simulink model "AirRefueling_Platform_IBVS"  (R2022b)
settings: Solver=ode4  StartTime=0.0  StopTime=60  FixedStep=0.01  RelTol=1e-5  AbsTol=1e-4  EnableMultiTasking=on
InitFcn:
  | F16_Init
values from neighbouring files (symbols this model uses):
  airSpeed = 393.72    [F16_Init.m]
  alpha0 = trimAlpha*180/pi    (= 6.62393794015)    [F16_Init.m]
  altitude = 9843    [F16_Init.m]
  b_ref = 30.0    (= 30)    [F16_Init.m]
  C2m = [C(1,:) ... (first row only)    [F16_Init.m]
  Cdr_ = 0.8    [hose_parameter4dock.mat]
  d_f_rc = [4.45;0;-3.81]    [F16_Init.m]
  d_pr_cam = d_pr_rc - d_cam_rc    [F16_Init.m]
  d_pr_rc = [8.2;0.45;-3.3]    [F16_Init.m]
  dLEF = 0    [F16_Init.m]
  dtheta10 = [0 0 0 0 0 0 0 0 0 0]    [hose_parameter4dock.mat]
  dtheta20 = [0 0 0 0 0 0 0 0 0 0]    [hose_parameter4dock.mat]
  fi_flag = 1    [F16_Init.m]
  height = 3000    [hose_parameter4dock.mat]
  k_reel = 0.5    [hose_parameter4dock.mat]
  Kc = [ ... (first row only)    [F16_Init.m]
  kd = 500    [hose_parameter4dock.mat]
  Ki = zeros(4,3)    [F16_Init.m]
  Kp = zeros(4,18)    [F16_Init.m]
  l0 = 1.44444444444    [hose_parameter4dock.mat]
  l1 = 2    [hose_parameter4dock.mat]
  l_density = 4.1    [hose_parameter4dock.mat]
  m0 = 5.92222222222    [hose_parameter4dock.mat]
  mass = 636.94    [F16_Init.m]
  Mdr = 29.5    [hose_parameter4dock.mat]
  N = 10    [hose_parameter4dock.mat]
  p0_rc = [-30.7;1;10]    [F16_Init.m]
  Rdr = 0.305    [hose_parameter4dock.mat]
  Rl = 0.0336    [hose_parameter4dock.mat]
  T_reel_initial = 1610    [hose_parameter4dock.mat]
  theta10 = [0.459903280115 0.432776206681 0.412025416789 0.390288667864 0.365355881715 0.340009787283 0.310854701374 0.281345523746 0.248396428993 0.214590627751]    [hose_parameter4dock.mat]
  theta20 = [0 0 0 0 0 0 0 0 0 0]    [hose_parameter4dock.mat]
  trim_ail = 0.00874607850103852    (= 0.00874607850104)    [F16_Init.m]
  trim_control = [trim_thrust;trim_ele;trim_ail;trim_rud]    [F16_Init.m]
  trim_ele = -2.97973164860638    (= -2.97973164861)    [F16_Init.m]
  trim_rud = 0.0680302158182712    (= 0.0680302158183)    [F16_Init.m]
  trim_state1 = [trim_state;0;0;0;0;0;0]    [F16_Init.m]
  trim_thrust = 2279.08519954656    (= 2279.08519955)    [F16_Init.m]
  visual_err = [0;0;0]    [F16_Init.m]
  vt0 = [120 0 0]    [hose_parameter4dock.mat]
undefined symbols (not defined in the file or in its folder): F, MIL, STD
libraries: etargetslib x11, dspnetwork x10, aerolibconvert2 x4, aerolibasang x4, simulink x2, aerolibatmos2 x2, aerolibwind2 x2, aerolibobsolete x2, aerolibadyn x1, aerolibanimutils x1, slrealtimeiplib x1
(part 2 of 3)

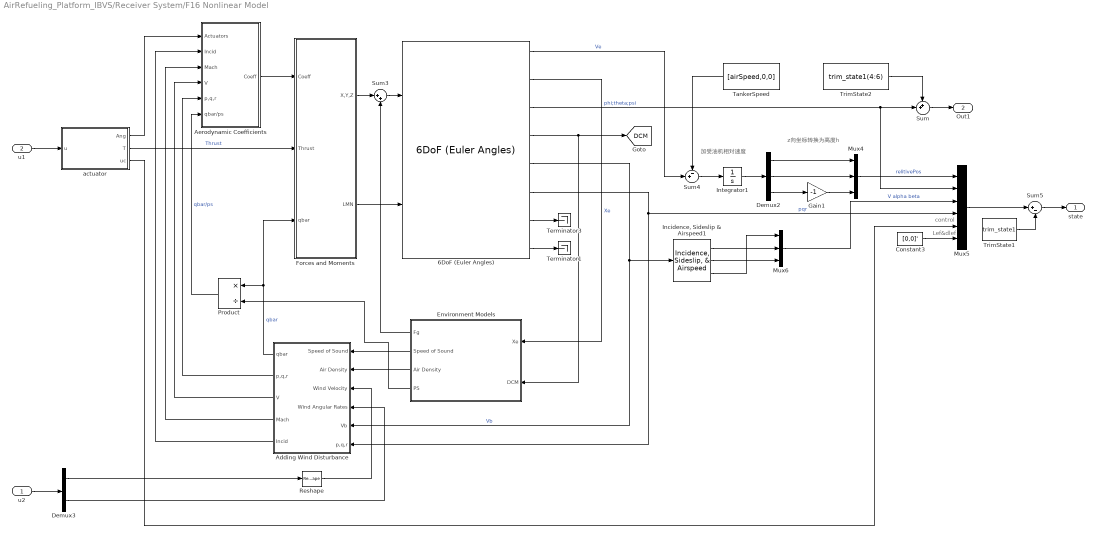
== system AirRefueling_Platform_IBVS/Receiver System/F16 Nonlinear Model ==
  note: 加受油机相对速度
  note: z向坐标转换为高度h
  note: Lef&dlef
  note: control
  u2 : Inport
  u1 : Inport  Port=2
  6DoF (Euler Angles) : aerolibobsolete/6DoF (Euler Angles)  units=English (Velocity in ft/s)  mtype=Fixed  rep=Euler Angles  xme_0=xyz_0  Vm_0=uvw_0  eul_0=Euler_0  pm_0=pqr_0  mass_0=mass  mass_e=0.5  mass_f=2.0  inertia=Inertia  inertia_e=eye(3)  inertia_f=2*eye(3)  k_quat=1.0
  Adding Wind Disturbance : Subsystem
  Aerodynamic Coefficients : Subsystem
  Constant3 : Constant  Value=[0,0]'
  Demux2 : Demux  Outputs=3
  Demux3 : Demux  Outputs=2
  Environment Models : Subsystem
  Forces and Moments : Subsystem
  Gain1 : Gain  Gain=-1
  "Incidence, Sideslip & Airspeed1" : aerolibasang/Incidence, Sideslip, & Airspeed
  Integrator1 : Integrator
  Mux4 : Mux  Inputs=3
  Mux5 : Mux  Inputs=6
  Mux6 : Mux  Inputs=3
  Product : Product  Inputs=*/  InputSameDT=on  SaturateOnIntegerOverflow=on  OutDataTypeStr=Inherit: Same as first input
  Reshape : Reshape
  Sum : Sum  Inputs=++|
  Sum3 : Sum  Inputs=|++  InputSameDT=on  SaturateOnIntegerOverflow=on  OutDataTypeStr=Inherit: Same as first input
  Sum4 : Sum  Inputs=-+|
  Sum5 : Sum  Inputs=|+-
  TankerSpeed : Constant  Value=[airSpeed,0,0]
  Terminator1 : Terminator
  Terminator3 : Terminator
  TrimState1 : Constant  Value=trim_state1
  TrimState2 : Constant  Value=trim_state1(4:6)
  actuator : Subsystem
  state : Outport
  Out1 : Outport  Port=2
  tag scope: DCM=global
  wires:
  6DoF (Euler Angles)/8 -> Terminator1/1
  6DoF (Euler Angles)/7 -> Terminator3/1
  6DoF (Euler Angles)/4 -> Environment Models/2(DCM), [DCM]
  Adding Wind Disturbance/5(Incid) -> Aerodynamic Coefficients/2(Incid)
  Aerodynamic Coefficients/1(Coeff) -> Forces and Moments/1(Coeff)
  Environment Models/2(Speed of Sound) -> Adding Wind Disturbance/1(Speed of Sound)
  Environment Models/3(Air Density) -> Adding Wind Disturbance/2(Air Density)
  Forces and Moments/2(LMN) -> 6DoF (Euler Angles)/2
  Adding Wind Disturbance/1(qbar) -> Forces and Moments/3(qbar), Product/1  "qbar"
  Forces and Moments/1(X,Y,Z) -> Sum3/1
  Sum3/1 -> 6DoF (Euler Angles)/1
  Environment Models/1(Fg) -> Sum3/2
  Adding Wind Disturbance/3(V) -> Aerodynamic Coefficients/4(V)
  Adding Wind Disturbance/4(Mach) -> Aerodynamic Coefficients/3(Mach)
  Adding Wind Disturbance/2("p,q,r ") -> Aerodynamic Coefficients/5(p,q,r)
  Environment Models/4(PS) -> Product/2
  Product/1 -> Aerodynamic Coefficients/6(qbar/ps)  "qbar/ps"
  u1/1 -> actuator/1(u)
  actuator/2(T) -> Forces and Moments/2(Thrust)  "Thrust"
  actuator/1(Ang) -> Aerodynamic Coefficients/1(Actuators)
  6DoF (Euler Angles)/3 -> Mux5/2, Sum/2  "phi;theta;psi"
  "Incidence, Sideslip & Airspeed1"/1 -> Mux6/2
  "Incidence, Sideslip & Airspeed1"/2 -> Mux6/3
  Mux6/1 -> Mux5/3  "V alpha beta"
  "Incidence, Sideslip & Airspeed1"/3 -> Mux6/1
  6DoF (Euler Angles)/6 -> Adding Wind Disturbance/6(p,q,r), Mux5/4  "pqr"
  6DoF (Euler Angles)/5 -> Adding Wind Disturbance/5(Vb), "Incidence, Sideslip & Airspeed1"/1  "Vb"
  Mux5/1 -> Sum5/1
  TrimState1/1 -> Sum5/2
  Sum5/1 -> state/1
  actuator/3(uc) -> Mux5/5
  Constant3/1 -> Mux5/6
  Demux2/2 -> Mux4/2
  Demux2/3 -> Gain1/1
  Mux4/1 -> Mux5/1  "relitivePos"
  Demux2/1 -> Mux4/1
  Gain1/1 -> Mux4/3
  Sum4/1 -> Integrator1/1
  Integrator1/1 -> Demux2/1
  6DoF (Euler Angles)/2 -> Environment Models/1(Xe)  "Xe"
  u2/1 -> Demux3/1
  Reshape/1 -> Adding Wind Disturbance/3(Wind Velocity)
  Demux3/1 -> Reshape/1
  Sum/1 -> Out1/1
  Demux3/2 -> Adding Wind Disturbance/4(Wind Angular Rates)
  TrimState2/1 -> Sum/1
  6DoF (Euler Angles)/1 -> Sum4/2  "Ve"
  TankerSpeed/1 -> Sum4/1

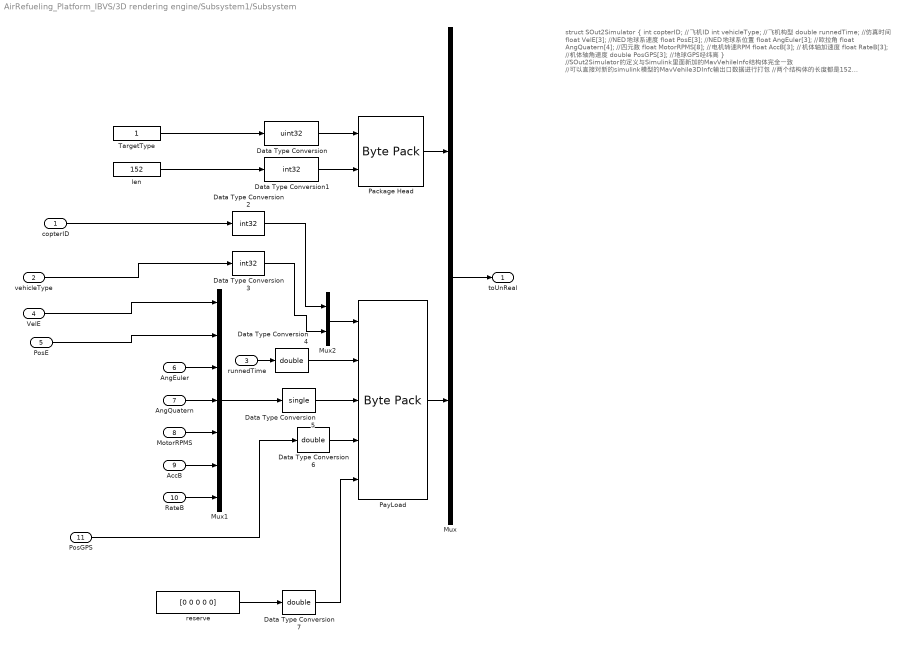
== system AirRefueling_Platform_IBVS/3D rendering engine/Subsystem1/Subsystem ==
  note: struct SOut2Simulator
      | {
      | int copterID; //飞机ID
      | int vehicleType; //飞机构型
      | double runnedTime; //仿真时间
      | float VelE[3]; //NED地球系速度
      | float PosE[3]; //NED地球系位置
      | float AngEuler[3]; //欧拉角
      | float AngQuatern[4]; //四元数
      | float MotorRPMS[8]; //电机转速RPM
      | float AccB[3]; //机体轴加速度
      | float RateB[3]; //机体轴角速度
      | double PosGPS[3]; //地球GPS经纬高
      | }
      |
      | //SOut2Simulator的定义与Simulink里面新加的MavVehileInfo结构体完全一致
      | //可以直接对新的simulink模型的MavVehile3DInfo输出口数据进行打包
      | //两个结构体的长度都是152
      | sizeof(SOut2Simulator) = sizeof(MavVehileInfo) = 152
      |
      | 打包封装的结构体为
      | typedef struct _netDataShort
      | {
      | TargetType tg; //这里目前随便填，写1即可 uint32
      | int len; //这个长度为传输结构体长度，目前是152
      | char payload[192]; //这里面前152位存放了SOut2Simulator结构体数据，后面的40位保留
      | }netDataShort;
      |
      | //UDP包的总长度为200
      | sizeof(netDataShort) = 200
      |
      | //发送的UDP端口号为：20010
  copterID : Inport  PortDimensions=1
  vehicleType : Inport  Port=2  PortDimensions=1
  runnedTime : Inport  Port=3  PortDimensions=1
  "VelE " : Inport  Port=4  PortDimensions=3
  PosE : Inport  Port=5  PortDimensions=3
  AngEuler : Inport  Port=6  PortDimensions=3
  AngQuatern : Inport  Port=7  PortDimensions=4
  MotorRPMS : Inport  Port=8  PortDimensions=8
  AccB : Inport  Port=9  PortDimensions=3
  RateB : Inport  Port=10  PortDimensions=3
  PosGPS : Inport  Port=11  PortDimensions=3
  Data Type Conversion : DataTypeConversion  OutDataTypeStr=uint32  SaturateOnIntegerOverflow=off  RndMeth=Floor
  Data Type Conversion1 : DataTypeConversion  OutDataTypeStr=int32  SaturateOnIntegerOverflow=off  RndMeth=Floor
  Data Type Conversion2 : DataTypeConversion  OutDataTypeStr=int32  SaturateOnIntegerOverflow=off  RndMeth=Floor
  Data Type Conversion3 : DataTypeConversion  OutDataTypeStr=int32  SaturateOnIntegerOverflow=off  RndMeth=Floor
  Data Type Conversion4 : DataTypeConversion  OutDataTypeStr=double  SaturateOnIntegerOverflow=off  RndMeth=Floor
  Data Type Conversion5 : DataTypeConversion  OutDataTypeStr=single  SaturateOnIntegerOverflow=off  RndMeth=Floor
  Data Type Conversion6 : DataTypeConversion  OutDataTypeStr=double  SaturateOnIntegerOverflow=off  RndMeth=Floor
  Data Type Conversion7 : DataTypeConversion  OutDataTypeStr=double  SaturateOnIntegerOverflow=off  RndMeth=Floor
  Mux : Mux  Inputs=2
  Mux1 : Mux  Inputs=7
  Mux2 : Mux  Inputs=2
  Package Head : etargetslib/Byte Pack  datatypes={'uint32','int32'}  byteAlign=4
  PayLoad : etargetslib/Byte Pack  datatypes={'int32','double','single','double','double'}  byteAlign=8
  TargetType : Constant  OutDataTypeStr=Inherit: Inherit via back propagation
  len : Constant  Value=152  OutDataTypeStr=Inherit: Inherit via back propagation
  reserve : Constant  Value=[0 0 0 0 0]  OutDataTypeStr=double
  toUnReal : Outport  VectorParamsAs1DForOutWhenUnconnected=off
  wires:
  runnedTime/1 -> Data Type Conversion4/1
  RateB/1 -> Mux1/7
  PayLoad/1 -> Mux/2
  "VelE "/1 -> Mux1/1
  Mux1/1 -> Data Type Conversion5/1
  PosGPS/1 -> Data Type Conversion6/1
  Package Head/1 -> Mux/1
  AccB/1 -> Mux1/6
  Mux/1 -> toUnReal/1
  MotorRPMS/1 -> Mux1/5
  AngQuatern/1 -> Mux1/4
  copterID/1 -> Data Type Conversion2/1
  len/1 -> Data Type Conversion1/1
  vehicleType/1 -> Data Type Conversion3/1
  PosE/1 -> Mux1/2
  TargetType/1 -> Data Type Conversion/1
  reserve/1 -> Data Type Conversion7/1
  Mux2/1 -> PayLoad/1
  AngEuler/1 -> Mux1/3
  Data Type Conversion5/1 -> PayLoad/3
  Data Type Conversion2/1 -> Mux2/1
  Data Type Conversion1/1 -> Package Head/2
  Data Type Conversion6/1 -> PayLoad/4
  Data Type Conversion/1 -> Package Head/1
  Data Type Conversion3/1 -> Mux2/2
  Data Type Conversion4/1 -> PayLoad/2
  Data Type Conversion7/1 -> PayLoad/5

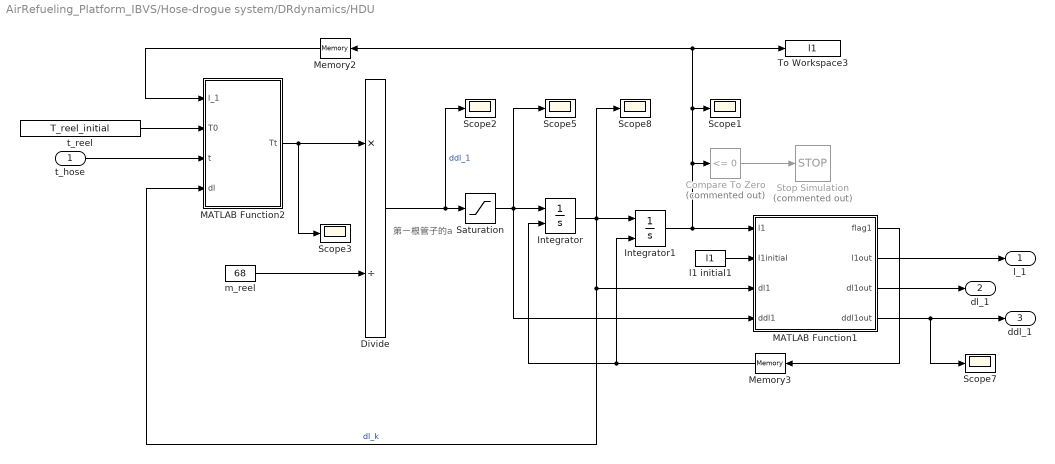
== system AirRefueling_Platform_IBVS/Hose-drogue system/DRdynamics/HDU ==
  note: 第一根管子的a
  t_hose : Inport
  Compare To Zero : simulink/Logic and Bit Operations/Compare To Zero  Commented=on  relop=<=  OutDataTypeStr=boolean
  Divide : Product  Inputs=*/
  Integrator : Integrator  ExternalReset=rising  UpperSaturationLimit=0.3  LowerSaturationLimit=-0.3
  Integrator1 : Integrator  ExternalReset=rising  InitialCondition=l1
  MATLAB Function1 : MATLAB Function  TreatAsAtomicUnit=on
  MATLAB Function2 : MATLAB Function  TreatAsAtomicUnit=on
  Memory2 : Memory  InitialCondition=l1
  Memory3 : Memory
  Saturation : Saturate  UpperLimit=3  LowerLimit=-3
  Scope{1..3,5,7..8} (6 alike) : Scope
  Stop Simulation : Stop  Commented=on
  To Workspace3 : ToWorkspace  VariableName=l1  SampleTime=-1
  l1 initial1 : Constant  Value=l1
  m_reel : Constant  Value=68
  t_reel : Constant  Value=T_reel_initial
  l_1 : Outport
  dl_1 : Outport  Port=2
  ddl_1 : Outport  Port=3
  wires:
  MATLAB Function2/1(Tt) -> Scope3/1, Divide/1
  m_reel/1 -> Divide/2
  Divide/1 -> Saturation/1, Scope2/1  "ddl_1"
  Integrator/1 -> Integrator1/1, MATLAB Function1/3(dl1), MATLAB Function2/4(dl), Scope8/1  "dl_k"
  Saturation/1 -> MATLAB Function1/4(ddl1), Integrator/1, Scope5/1
  t_reel/1 -> MATLAB Function2/2(T0)
  Compare To Zero/1 -> Stop Simulation/1
  l1 initial1/1 -> MATLAB Function1/2(l1initial)
  MATLAB Function1/4(ddl1out) -> Scope7/1, ddl_1/1
  MATLAB Function1/1(flag1) -> Memory3/1
  Memory2/1 -> MATLAB Function2/1(l_1)
  Memory3/1 -> Integrator/2, Integrator1/2
  Integrator1/1 -> MATLAB Function1/1(l1), Compare To Zero/1, To Workspace3/1, Memory2/1, Scope1/1
  MATLAB Function1/2(l1out) -> l_1/1
  MATLAB Function1/3(dl1out) -> dl_1/1
  t_hose/1 -> MATLAB Function2/3(t)

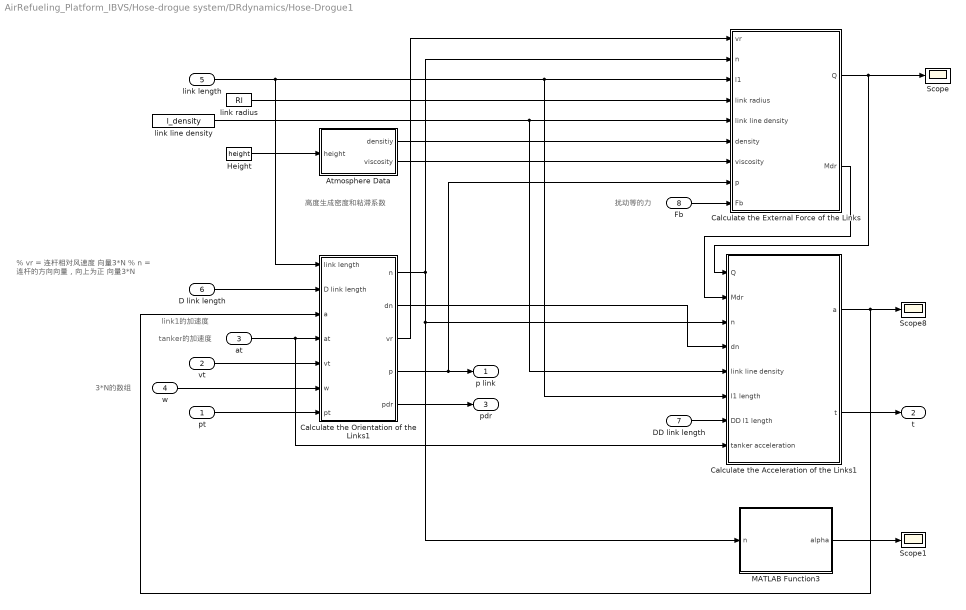
== system AirRefueling_Platform_IBVS/Hose-drogue system/DRdynamics/Hose-Drogue1 ==
  note: % vr = 连杆相对风速度 向量3*N
      | % n = 连杆的方向向量，向上为正 向量3*N
  note: link1的加速度
  note: tanker的加速度
  note: 3*N的数组
  note: 扰动等的力
  note: 高度生成密度和粘滞系数
  pt : Inport
  vt : Inport  Port=2
  at : Inport  Port=3
  w : Inport  Port=4
  link length : Inport  Port=5
  D link length : Inport  Port=6
  DD link length : Inport  Port=7
  Fb : Inport  Port=8
  Atmosphere Data : Subsystem
  Calculate the Acceleration of the Links1 : Subsystem
  Calculate the External Force of the Links : Subsystem
  Calculate the Orientation of the Links1 : Subsystem
  Height : Constant  Value=height
  MATLAB Function3 : MATLAB Function  TreatAsAtomicUnit=on
  Scope : Scope
  Scope1 : Scope
  Scope8 : Scope
  link line density : Constant  Value=l_density
  link radius : Constant  Value=Rl
  p link : Outport
  t : Outport  Port=2
  pdr : Outport  Port=3
  wires:
  Height/1 -> Atmosphere Data/1(height)
  Atmosphere Data/1(densitiy) -> Calculate the External Force of the Links/6(density)
  Atmosphere Data/2(viscosity) -> Calculate the External Force of the Links/7(viscosity)
  link radius/1 -> Calculate the External Force of the Links/4(link radius)
  link line density/1 -> Calculate the External Force of the Links/5(link line density), Calculate the Acceleration of the Links1/5(link line density)
  Calculate the External Force of the Links/1(Q) -> Scope/1, Calculate the Acceleration of the Links1/1(Q)
  Calculate the Orientation of the Links1/1(n) -> Calculate the External Force of the Links/2(n), MATLAB Function3/1(n), Calculate the Acceleration of the Links1/3(n)
  Calculate the Orientation of the Links1/2(dn) -> Calculate the Acceleration of the Links1/4(dn)
  Calculate the External Force of the Links/2(Mdr) -> Calculate the Acceleration of the Links1/2(Mdr)
  at/1 -> Calculate the Orientation of the Links1/4(at), Calculate the Acceleration of the Links1/8("tanker acceleration ")
  Calculate the Orientation of the Links1/3(vr) -> Calculate the External Force of the Links/1(vr)
  w/1 -> Calculate the Orientation of the Links1/6(w)
  Calculate the Acceleration of the Links1/1(a) -> Calculate the Orientation of the Links1/3(a), Scope8/1
  Calculate the Orientation of the Links1/4(p) -> Calculate the External Force of the Links/8(p), p link/1
  pt/1 -> Calculate the Orientation of the Links1/7(pt)
  vt/1 -> Calculate the Orientation of the Links1/5(vt)
  Calculate the Acceleration of the Links1/2(t) -> t/1
  link length/1 -> Calculate the Orientation of the Links1/1(link length), Calculate the External Force of the Links/3(l1), Calculate the Acceleration of the Links1/6(l1 length)
  D link length/1 -> Calculate the Orientation of the Links1/2(D link length)
  DD link length/1 -> Calculate the Acceleration of the Links1/7(DD l1 length)
  Fb/1 -> Calculate the External Force of the Links/9(Fb)
  MATLAB Function3/1(alpha) -> Scope1/1
  Calculate the Orientation of the Links1/5(pdr) -> pdr/1

== system AirRefueling_Platform_IBVS/Receiver System/F16 Nonlinear Model/Adding Wind Disturbance ==
  Speed of Sound : Inport
  Air Density : Inport  Port=2
  Wind Velocity : Inport  Port=3  PortDimensions=3
  Wind Angular Rates : Inport  Port=4  PortDimensions=3
  Vb : Inport  Port=5  PortDimensions=3
  p,q,r : Inport  Port=6  PortDimensions=3
  Dynamic Pressure : aerolibasang/Dynamic Pressure
  "Incidence, Sideslip & Airspeed" : aerolibasang/Incidence, Sideslip, & Airspeed
  Mach Number : aerolibasang/Mach Number
  Mux : Mux  Inputs=2
  Sum : Sum  Inputs=|+-  InputSameDT=on  SaturateOnIntegerOverflow=on  OutDataTypeStr=Inherit: Same as first input
  Sum1 : Sum  Inputs=|++  InputSameDT=on  SaturateOnIntegerOverflow=on  OutDataTypeStr=Inherit: Same as first input
  qbar : Outport  InitialOutput=0
  "p,q,r " : Outport  Port=2
  V : Outport  Port=3
  Mach : Outport  Port=4
  Incid : Outport  Port=5
  wires:
  "Incidence, Sideslip & Airspeed"/3 -> V/1
  Dynamic Pressure/1 -> qbar/1
  Air Density/1 -> Dynamic Pressure/2
  Mach Number/1 -> Mach/1
  Sum/1 -> Dynamic Pressure/1, Mach Number/1, "Incidence, Sideslip & Airspeed"/1
  Vb/1 -> Sum/1
  Speed of Sound/1 -> Mach Number/2
  Wind Velocity/1 -> Sum/2
  "Incidence, Sideslip & Airspeed"/2 -> Mux/2  "Beta"
  Mux/1 -> Incid/1
  "Incidence, Sideslip & Airspeed"/1 -> Mux/1  "Alpha"
  p,q,r/1 -> Sum1/1
  Wind Angular Rates/1 -> Sum1/2
  Sum1/1 -> "p,q,r "/1

== system AirRefueling_Platform_IBVS/Receiver System/F16 Nonlinear Model/Aerodynamic Coefficients ==
  Actuators : Inport
  Incid : Inport  Port=2
  Mach : Inport  Port=3
  V : Inport  Port=4
  p,q,r : Inport  Port=5
  qbar/ps : Inport  Port=6
  Angle Conversion : aerolibconvert2/Angle Conversion  IU=rad  OU=deg
  Interpreted MATLAB Function : MATLABFcn  MATLABFcn=F16Coef1  OutputDimensions=6
  Leading Edge Flap : Subsystem
  Mux : Mux  Inputs=6
  Terminator2 : Terminator
  alpha : Selector  InputPortWidth=2  IndexOptions=Index vector (dialog)  Indices=1  OutputSizes=1
  flag : Constant  Value=fi_flag
  Coeff : Outport  InitialOutput=0
  wires:
  Angle Conversion/1 -> alpha/1, Mux/2
  Incid/1 -> Angle Conversion/1
  qbar/ps/1 -> Leading Edge Flap/2(qbar/ps)
  alpha/1 -> Leading Edge Flap/1(alpha)
  V/1 -> Mux/1
  p,q,r/1 -> Mux/3
  Actuators/1 -> Mux/4
  flag/1 -> Mux/5
  Mach/1 -> Terminator2/1
  Interpreted MATLAB Function/1 -> Coeff/1
  Mux/1 -> Interpreted MATLAB Function/1
  Leading Edge Flap/1(delta_lef (deg)) -> Mux/6

== system AirRefueling_Platform_IBVS/Receiver System/F16 Nonlinear Model/Environment Models ==
  Xe : Inport  PortDimensions=3
  DCM : Inport  Port=2
  COESA Atmosphere Model : aerolibatmos2/COESA Atmosphere Model  units=English (Velocity in ft/s)  spec=1976 COESA-extended U.S. Standard Atmosphere  model=Profile  profile_var=High temperature  profile_percent=10%  profile_alt=5 km (16404 ft)  envelope_var=High temperature  envelope_percent=1%  action=None
  Clock : Clock
  Constant : Constant  Value=mass
  Gravity in Earth Axes : Gain  Commented=on  Gain=mass  SaturateOnIntegerOverflow=on  OutDataTypeStr=Inherit: Same as input  ParamDataTypeStr=Inherit: Same as input
  Height : Selector  InputPortWidth=3  IndexOptions=Index vector (dialog)  Indices=[3]  OutputSizes=1
  Inertial to Body : Product  Multiplication=Matrix(*)  InputSameDT=on  SaturateOnIntegerOverflow=on  OutDataTypeStr=Inherit: Same as first input
  Latitude : Constant  Value=0
  Mux : Mux  Inputs=3
  Product6 : Product  Inputs=**  InputSameDT=on  SaturateOnIntegerOverflow=on  OutDataTypeStr=Inherit: Same as first input
  Reshape : Reshape
  Terminator : Terminator
  "WGS84 Gravity Model " : aerolibobsolete/WGS84 Gravity Model   model=WGS84 Taylor Series  units=English  no_atmos=on  precessing=on  jd_loc=off  month=October  day=10  year=2004  no_centrifugal=on  action=None
  mass variable : MATLAB Function  TreatAsAtomicUnit=on
  r2d5 : Gain  Gain=1715  SaturateOnIntegerOverflow=on  OutDataTypeStr=Inherit: Same as input  ParamDataTypeStr=Inherit: Same as input
  z-->h : Abs
  Fg : Outport  InitialOutput=0
  Speed of Sound : Outport  Port=2  InitialOutput=0
  Air Density : Outport  Port=3  InitialOutput=0
  PS : Outport  Port=4
  wires:
  Reshape/1 -> Inertial to Body/2
  Mux/1 -> "WGS84 Gravity Model "/1
  z-->h/1 -> Mux/3, COESA Atmosphere Model/1
  COESA Atmosphere Model/2 -> Speed of Sound/1
  COESA Atmosphere Model/3 -> Terminator/1
  Height/1 -> z-->h/1
  Xe/1 -> Height/1
  Latitude/1 -> Mux/2, Mux/1
  "WGS84 Gravity Model "/1 -> mass variable/1(g)
  mass variable/1(y) -> Reshape/1
  DCM/1 -> Inertial to Body/1
  Inertial to Body/1 -> Fg/1
  COESA Atmosphere Model/4 -> Product6/2, Air Density/1
  COESA Atmosphere Model/1 -> r2d5/1
  Product6/1 -> PS/1
  r2d5/1 -> Product6/1
  Clock/1 -> mass variable/3(time)
  Constant/1 -> mass variable/2(mass)

== system AirRefueling_Platform_IBVS/Receiver System/F16 Nonlinear Model/Forces and Moments ==
  Coeff : Inport
  Thrust : Inport  Port=2
  qbar : Inport  Port=3
  "Aerodynamic Forces and Moments " : aerolibadyn/Aerodynamic Forces and Moments   inputAxes=Body  outputForceAxes=Body  outputMomentAxes=Body  S=S_ref  b=b_ref  cbar=d_ref
  Center of Gravity : Constant  Value=[-0 0 0]
  Center of Pressure : Constant  Value=[-0 0 0]
  Sum : Sum  Inputs=++|  InputSameDT=on  SaturateOnIntegerOverflow=on  OutDataTypeStr=Inherit: Same as first input
  X,Y,Z : Outport  InitialOutput=0
  LMN : Outport  Port=2  InitialOutput=0
  wires:
  Center of Pressure/1 -> "Aerodynamic Forces and Moments "/4
  Center of Gravity/1 -> "Aerodynamic Forces and Moments "/3
  "Aerodynamic Forces and Moments "/1 -> Sum/2
  "Aerodynamic Forces and Moments "/2 -> LMN/1
  Sum/1 -> X,Y,Z/1
  Thrust/1 -> Sum/1
  qbar/1 -> "Aerodynamic Forces and Moments "/2
  Coeff/1 -> "Aerodynamic Forces and Moments "/1

== system AirRefueling_Platform_IBVS/Receiver System/F16 Nonlinear Model/actuator ==
  u : Inport
  Aileron Actuator : Subsystem
  Demux : Demux
  Elevator Actuator : Subsystem
  Mux : Mux  Inputs=2
  Mux1 : Mux  Inputs=3
  Mux2 : Mux  Inputs=3
  Rudder Actuator : Subsystem
  Thrust Model : Subsystem
  Ty : Constant  Value=0
  Tz : Constant  Value=0
  Ang : Outport
  T : Outport  Port=2
  uc : Outport  Port=3
  wires:
  u/1 -> Demux/1
  Mux2/1 -> Ang/1, Mux/2
  Thrust Model/1(T) -> Mux/1, Mux1/1  "Tx"
  Ty/1 -> Mux1/2
  Tz/1 -> Mux1/3
  Mux1/1 -> T/1
  Mux/1 -> uc/1
  Demux/1 -> Thrust Model/1(delta_t)
  Elevator Actuator/1(el) -> Mux2/1  "el"
  Aileron Actuator/1(ail) -> Mux2/2  "ail"
  Rudder Actuator/1(rud) -> Mux2/3  "rud"
  Demux/2 -> Elevator Actuator/1(delta_e)
  Demux/3 -> Aileron Actuator/1(delta_a)
  Demux/4 -> Rudder Actuator/1(delta_r)

== system AirRefueling_Platform_IBVS/Hose-drogue system/DRdynamics/Hose-Drogue1/Atmosphere Data ==
  height : Inport
  1-D Lookup Table : Lookup_n-D  NumberOfTableDimensions=1  BreakpointsForDimension1=[0,1000,2000,3000,4000,5000,6000,7000,8000,9000,10000]  Table=[1.789e-05,1.749e-05,1.717e-05,1.684e-05,1.652e-05,1.619e-05,1.586e-05,1.552e-05,1.517e-05,1.482e-05,1.447e-05]  RndMeth=Simplest
  COESA Atmosphere Model : aerolibatmos2/COESA Atmosphere Model  units=Metric (MKS)  spec=MIL-STD-210C  model=Profile  profile_var=High temperature  profile_percent=1%  profile_alt=5 km (16404 ft)  envelope_var=High temperature  envelope_percent=1%  action=Warning
  Terminator : Terminator
  Terminator1 : Terminator
  Terminator2 : Terminator
  densitiy : Outport
  viscosity : Outport  Port=2
  wires:
  COESA Atmosphere Model/4 -> densitiy/1
  height/1 -> 1-D Lookup Table/1, COESA Atmosphere Model/1
  COESA Atmosphere Model/1 -> Terminator/1
  COESA Atmosphere Model/2 -> Terminator1/1
  COESA Atmosphere Model/3 -> Terminator2/1
  1-D Lookup Table/1 -> viscosity/1

== system AirRefueling_Platform_IBVS/Hose-drogue system/DRdynamics/Hose-Drogue1/Calculate the Acceleration of the Links1 ==
  note: 得到第一根杆子的拉力
  note: 计算出第一根杆子的外力
  Q : Inport
  Mdr : Inport  Port=2
  n : Inport  Port=3
  dn : Inport  Port=4
  link line density : Inport  Port=5
  l1 length : Inport  Port=6
  DD l1 length : Inport  Port=7
  "tanker acceleration " : Inport  Port=8
  IC : InitialCondition  Value=0
  MATLAB Function : MATLAB Function  TreatAsAtomicUnit=on
  MATLAB Function2 : MATLAB Function  TreatAsAtomicUnit=on
  MATLAB Function3 : MATLAB Function  TreatAsAtomicUnit=on
  MATLAB Function4 : MATLAB Function  TreatAsAtomicUnit=on
  Product : Product
  a : Outport
  t : Outport  Port=2
  wires:
  n/1 -> MATLAB Function4/1(n), MATLAB Function3/3(n), MATLAB Function/1(n)
  Product/1 -> MATLAB Function3/4(m1), MATLAB Function4/4(m1), MATLAB Function/2(m1)  "l1 mass"
  Q/1 -> MATLAB Function4/3(Q), MATLAB Function3/2(Q)
  DD l1 length/1 -> MATLAB Function4/6(ddl1)
  "tanker acceleration "/1 -> MATLAB Function4/7(a0)
  dn/1 -> MATLAB Function4/2(dn)
  l1 length/1 -> MATLAB Function4/5(l1), Product/2
  link line density/1 -> Product/1
  MATLAB Function/1(T) -> MATLAB Function2/1(T)
  MATLAB Function4/1(q) -> MATLAB Function2/2(q)
  MATLAB Function2/2(t) -> IC/1
  Mdr/1 -> MATLAB Function3/5(Mdr)
  MATLAB Function3/1(a) -> a/1
  MATLAB Function2/1(t0) -> t/1
  IC/1 -> MATLAB Function3/1(t)

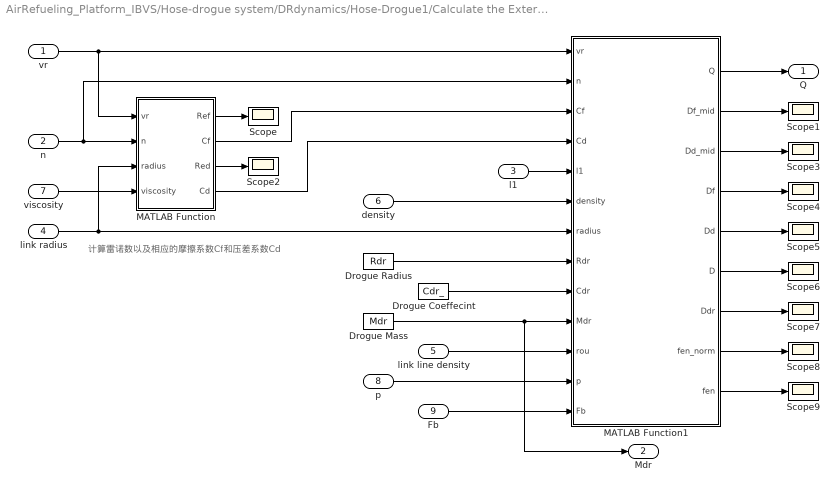
== system AirRefueling_Platform_IBVS/Hose-drogue system/DRdynamics/Hose-Drogue1/Calculate the External Force of the Links ==
  note: 计算雷诺数以及相应的摩擦系数Cf和压差系数Cd
  vr : Inport
  n : Inport  Port=2
  l1 : Inport  Port=3
  link radius : Inport  Port=4
  link line density : Inport  Port=5
  density : Inport  Port=6
  viscosity : Inport  Port=7
  p : Inport  Port=8
  Fb : Inport  Port=9
  Drogue Coeffecint : Constant  Value=Cdr_
  Drogue Mass : Constant  Value=Mdr
  Drogue Radius : Constant  Value=Rdr
  MATLAB Function : MATLAB Function  TreatAsAtomicUnit=on
  MATLAB Function1 : MATLAB Function  TreatAsAtomicUnit=on
  Scope{,1..9} (10 alike) : Scope
  Q : Outport
  Mdr : Outport  Port=2
  wires:
  MATLAB Function/1(Ref) -> Scope/1
  MATLAB Function/3(Red) -> Scope2/1
  MATLAB Function1/1(Q) -> Q/1
  vr/1 -> MATLAB Function/1(vr), MATLAB Function1/1(vr)
  n/1 -> MATLAB Function1/2(n), MATLAB Function/2(n)
  link radius/1 -> MATLAB Function/3(radius), MATLAB Function1/7(radius)
  viscosity/1 -> MATLAB Function/4(viscosity)
  density/1 -> MATLAB Function1/6(density)
  Drogue Radius/1 -> MATLAB Function1/8(Rdr)
  Drogue Coeffecint/1 -> MATLAB Function1/9(Cdr)
  Drogue Mass/1 -> Mdr/1, MATLAB Function1/10(Mdr)
  link line density/1 -> MATLAB Function1/11(rou)
  MATLAB Function1/2(Df_mid) -> Scope1/1
  MATLAB Function1/3(Dd_mid) -> Scope3/1
  MATLAB Function1/4(Df) -> Scope4/1
  MATLAB Function1/5(Dd) -> Scope5/1
  MATLAB Function1/6(D) -> Scope6/1
  MATLAB Function1/7(Ddr) -> Scope7/1
  MATLAB Function/2(Cf) -> MATLAB Function1/3(Cf)
  MATLAB Function/4(Cd) -> MATLAB Function1/4(Cd)
  p/1 -> MATLAB Function1/12(p)
  l1/1 -> MATLAB Function1/5(l1)
  Fb/1 -> MATLAB Function1/13(Fb)
  MATLAB Function1/8(fen_norm) -> Scope8/1
  MATLAB Function1/9(fen) -> Scope9/1

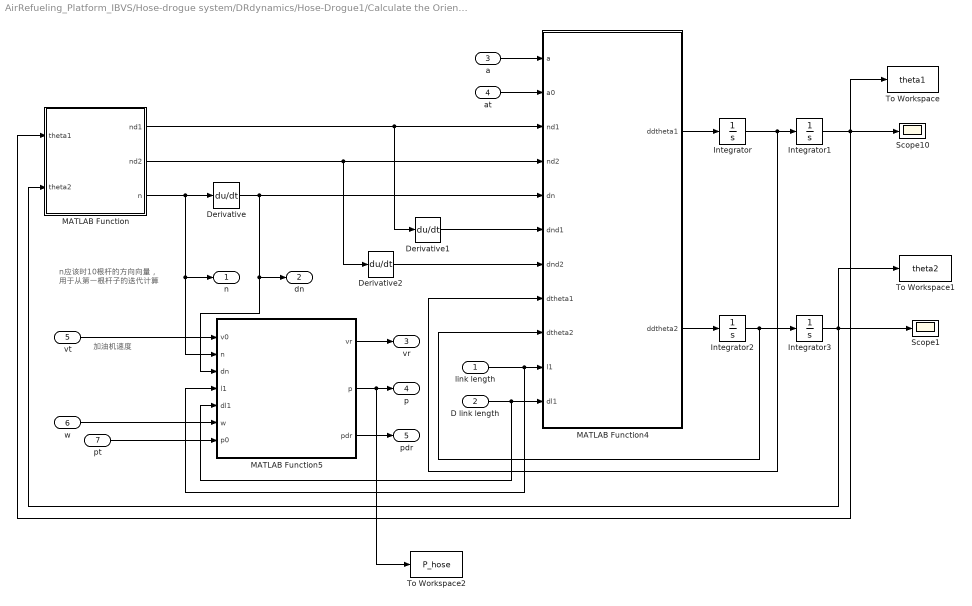
== system AirRefueling_Platform_IBVS/Hose-drogue system/DRdynamics/Hose-Drogue1/Calculate the Orientation of the Links1 ==
  note: n应该时10根杆的方向向量，
      | 用于从第一根杆子的迭代计算
  note: 加油机速度
  link length : Inport
  D link length : Inport  Port=2
  a : Inport  Port=3
  at : Inport  Port=4
  vt : Inport  Port=5
  w : Inport  Port=6
  pt : Inport  Port=7
  Derivative : Derivative
  Derivative1 : Derivative
  Derivative2 : Derivative
  Integrator : Integrator  InitialCondition=dtheta10
  Integrator1 : Integrator  InitialCondition=theta10
  Integrator2 : Integrator  InitialCondition=dtheta20
  Integrator3 : Integrator  InitialCondition=theta20
  MATLAB Function : MATLAB Function  TreatAsAtomicUnit=on
  MATLAB Function4 : MATLAB Function  TreatAsAtomicUnit=on
  MATLAB Function5 : MATLAB Function  TreatAsAtomicUnit=on
  Scope1 : Scope
  Scope10 : Scope
  To Workspace : ToWorkspace  VariableName=theta1  SampleTime=-1
      settings: Save2DSignal=2-D array (concatenate along first dimension)
  To Workspace1 : ToWorkspace  VariableName=theta2  SampleTime=-1
      settings: Save2DSignal=2-D array (concatenate along first dimension)
  To Workspace2 : ToWorkspace  VariableName=P_hose  SampleTime=-1
  n : Outport
  dn : Outport  Port=2
  vr : Outport  Port=3
  p : Outport  Port=4
  pdr : Outport  Port=5
  wires:
  Integrator1/1 -> To Workspace/1, MATLAB Function/1(theta1), Scope10/1
  Integrator3/1 -> To Workspace1/1, MATLAB Function/2(theta2), Scope1/1
  MATLAB Function/3(n) -> MATLAB Function5/2(n), n/1, Derivative/1
  Integrator/1 -> MATLAB Function4/8(dtheta1), Integrator1/1
  Integrator2/1 -> MATLAB Function4/9(dtheta2), Integrator3/1
  Derivative1/1 -> MATLAB Function4/6(dnd1)
  Derivative2/1 -> MATLAB Function4/7(dnd2)
  MATLAB Function4/2(ddtheta2) -> Integrator2/1
  link length/1 -> MATLAB Function4/10(l1), MATLAB Function5/4(l1)
  D link length/1 -> MATLAB Function5/5(dl1), MATLAB Function4/11(dl1)
  a/1 -> MATLAB Function4/1(a)
  at/1 -> MATLAB Function4/2(a0)
  vt/1 -> MATLAB Function5/1(v0)
  w/1 -> MATLAB Function5/6(w)
  MATLAB Function5/1(vr) -> vr/1
  pt/1 -> MATLAB Function5/7(p0)
  MATLAB Function/1(nd1) -> Derivative1/1, MATLAB Function4/3(nd1)
  MATLAB Function/2(nd2) -> Derivative2/1, MATLAB Function4/4(nd2)
  Derivative/1 -> MATLAB Function5/3(dn), dn/1, MATLAB Function4/5(dn)
  MATLAB Function5/3(pdr) -> pdr/1
  MATLAB Function5/2(p) -> To Workspace2/1, p/1
  MATLAB Function4/1(ddtheta1) -> Integrator/1

== system AirRefueling_Platform_IBVS/Receiver System/F16 Nonlinear Model/Aerodynamic Coefficients/Leading Edge Flap ==
  note: see NASA Technical Paper 1538, p34
  note: Initialize LF_state with -alpha0 value in degrees!!!!
  alpha : Inport
  qbar/ps : Inport  Port=2
  Gain : Gain  Gain=2  SaturateOnIntegerOverflow=on  OutDataTypeStr=Inherit: Same as input  ParamDataTypeStr=Inherit: Same as input
  Gain1 : Gain  Gain=7.25  SaturateOnIntegerOverflow=on  OutDataTypeStr=Inherit: Same as input  ParamDataTypeStr=Inherit: Same as input
  Gain2 : Gain  Gain=1.38  SaturateOnIntegerOverflow=on  OutDataTypeStr=Inherit: Same as input  ParamDataTypeStr=Inherit: Same as input
  LEF Actuator : Subsystem
  LF_state : Integrator  InitialCondition=-alpha0
  Sum : Sum  Inputs=-|+|+  InputSameDT=on  SaturateOnIntegerOverflow=on  OutDataTypeStr=Inherit: Same as first input
  Sum1 : Sum  Inputs=|+-  InputSameDT=on  SaturateOnIntegerOverflow=on  OutDataTypeStr=Inherit: Same as first input
  Sum2 : Sum  Inputs=++|  InputSameDT=on  SaturateOnIntegerOverflow=on  OutDataTypeStr=Inherit: Same as first input
  coeff1 : Constant  Value=1.45
  lef Saturation : Saturate  UpperLimit=25  LowerLimit=0
  r2d6 : Gain  Gain=9.05  SaturateOnIntegerOverflow=on  OutDataTypeStr=Inherit: Same as input  ParamDataTypeStr=Inherit: Same as input
  delta_lef (deg) : Outport
  wires:
  Sum1/1 -> Gain1/1
  Gain1/1 -> LF_state/1
  Gain/1 -> Sum2/1
  Gain2/1 -> Sum/2
  coeff1/1 -> Sum/3
  Sum2/1 -> Sum1/2, Gain2/1
  LF_state/1 -> Sum2/2
  alpha/1 -> Sum1/1, Gain/1
  qbar/ps/1 -> r2d6/1
  r2d6/1 -> Sum/1
  lef Saturation/1 -> delta_lef (deg)/1
  Sum/1 -> LEF Actuator/1(dlef)
  LEF Actuator/1(LEF) -> lef Saturation/1

== system AirRefueling_Platform_IBVS/Receiver System/F16 Nonlinear Model/actuator/Aileron Actuator ==
  delta_a : Inport
  Command Saturation : Saturate  UpperLimit=21.5  LowerLimit=-21.5
  Gain : Gain  Gain=20.2  SaturateOnIntegerOverflow=on  OutDataTypeStr=Inherit: Same as input  ParamDataTypeStr=Inherit: Same as input
  "Integrator " : Integrator  InitialCondition=trim_ail  UpperSaturationLimit=21.5  LowerSaturationLimit=-21.5
  Rate Saturation : Saturate  UpperLimit=80  LowerLimit=-80
  Sum : Sum  Inputs=|+-  InputSameDT=on  SaturateOnIntegerOverflow=on  OutDataTypeStr=Inherit: Same as first input
  ail : Outport
  wires:
  delta_a/1 -> Command Saturation/1
  "Integrator "/1 -> ail/1, Sum/2
  Sum/1 -> Gain/1
  Gain/1 -> Rate Saturation/1
  Command Saturation/1 -> Sum/1
  Rate Saturation/1 -> "Integrator "/1

== system AirRefueling_Platform_IBVS/Receiver System/F16 Nonlinear Model/actuator/Elevator Actuator ==
  delta_e : Inport
  Command Saturation : Saturate  UpperLimit=25  LowerLimit=-25
  Gain : Gain  Gain=20.2  SaturateOnIntegerOverflow=on  OutDataTypeStr=Inherit: Same as input  ParamDataTypeStr=Inherit: Same as input
  "Integrator " : Integrator  InitialCondition=trim_ele  UpperSaturationLimit=25  LowerSaturationLimit=-25
  Rate Saturation : Saturate  UpperLimit=60  LowerLimit=-60
  Sum : Sum  Inputs=|+-  InputSameDT=on  SaturateOnIntegerOverflow=on  OutDataTypeStr=Inherit: Same as first input
  el : Outport
  wires:
  delta_e/1 -> Command Saturation/1
  Command Saturation/1 -> Sum/1
  Sum/1 -> Gain/1
  Gain/1 -> Rate Saturation/1
  "Integrator "/1 -> el/1, Sum/2
  Rate Saturation/1 -> "Integrator "/1

== system AirRefueling_Platform_IBVS/Receiver System/F16 Nonlinear Model/actuator/Rudder Actuator ==
  delta_r : Inport
  Command Saturation : Saturate  UpperLimit=30  LowerLimit=-30
  Gain : Gain  Gain=20.2  SaturateOnIntegerOverflow=on  OutDataTypeStr=Inherit: Same as input  ParamDataTypeStr=Inherit: Same as input
  "Integrator " : Integrator  InitialCondition=trim_rud  UpperSaturationLimit=30  LowerSaturationLimit=-30
  Rate Saturation : Saturate  UpperLimit=120  LowerLimit=-120
  Sum : Sum  Inputs=|+-  InputSameDT=on  SaturateOnIntegerOverflow=on  OutDataTypeStr=Inherit: Same as first input
  rud : Outport
  wires:
  "Integrator "/1 -> rud/1, Sum/2
  Sum/1 -> Gain/1
  delta_r/1 -> Command Saturation/1
  Rate Saturation/1 -> "Integrator "/1
  Gain/1 -> Rate Saturation/1
  Command Saturation/1 -> Sum/1

== system AirRefueling_Platform_IBVS/Receiver System/F16 Nonlinear Model/actuator/Thrust Model ==
  delta_t : Inport
  Command Saturation : Saturate  UpperLimit=19000  LowerLimit=1000
  Gain : Gain  SaturateOnIntegerOverflow=on  OutDataTypeStr=Inherit: Same as input  ParamDataTypeStr=Inherit: Same as input
  "Integrator " : Integrator  InitialCondition=trim_thrust  UpperSaturationLimit=30  LowerSaturationLimit=-30
  Rate Saturation : Saturate  UpperLimit=10000  LowerLimit=-10000
  Sum : Sum  Inputs=|+-  InputSameDT=on  SaturateOnIntegerOverflow=on  OutDataTypeStr=Inherit: Same as first input
  T : Outport
  wires:
  delta_t/1 -> Command Saturation/1
  Gain/1 -> Rate Saturation/1
  "Integrator "/1 -> T/1, Sum/2
  Command Saturation/1 -> Sum/1
  Sum/1 -> Gain/1
  Rate Saturation/1 -> "Integrator "/1

== system AirRefueling_Platform_IBVS/Receiver System/F16 Nonlinear Model/Aerodynamic Coefficients/Leading Edge Flap/LEF Actuator ==
  dlef : Inport
  Command Saturation : Saturate  UpperLimit=25  LowerLimit=0
  Gain3 : Gain  Gain=1/0.136  SaturateOnIntegerOverflow=on  OutDataTypeStr=Inherit: Same as input  ParamDataTypeStr=Inherit: Same as input
  "Integrator " : Integrator  InitialCondition=dLEF  UpperSaturationLimit=21.5  LowerSaturationLimit=-21.5
  Rate Saturation : Saturate  UpperLimit=25  LowerLimit=-25
  Sum3 : Sum  Inputs=|+-  InputSameDT=on  SaturateOnIntegerOverflow=on  OutDataTypeStr=Inherit: Same as first input
  LEF : Outport
  wires:
  Gain3/1 -> Rate Saturation/1
  Rate Saturation/1 -> "Integrator "/1
  "Integrator "/1 -> LEF/1, Sum3/2
  Sum3/1 -> Gain3/1
  dlef/1 -> Command Saturation/1
  Command Saturation/1 -> Sum3/1

== matlab function AirRefueling_Platform_IBVS/SimToUE ==
  data: y output; PosRc input; PosTb1 input; Pos_dr2tx output
function [y,Pos_dr2tx] = SimToVR(PosRc,PosTb1)
%#codegen

%%函数名：SimToVR
%%用途  ：将软管锥套坐标输出转换为VR输入
%%输入  ：PosPr - 受油机坐标， PlsTb - 软管坐标数据
%%输出  ：VrPos - 软管和受油机VR位置，VrAngle - 旋转角度输出
%%作者  ：戴训华
%%时间  ：2014/3/19

Pos_rc2tx = PosRc(4:6);
% add PosPr1(4:6)存储的是受油机的姿态  模型中在输出姿态[phi, theta, psai]后加上了trim_state1=[0;0.1156,0],这里又给减掉了
% 无人机先绕机体系 z 轴旋转 ψ \psiψ，再绕机体系 y 轴旋转 θ \thetaθ，最后绕机体系 x 轴旋转 ϕ \phiϕ，[yaw,pitch,roll]
% AttitudeRecei = [PosPr1(4);-PosPr1(6);PosPr1(5)-0.115609];
AttitudeRecei = [0;0.1156;0];
PosTb = PosTb1(1:60);

% 这个不用 用的是通过最后一根杆子生成锥套的方法
PosDr = PosTb1(61:63);

% 这里是20根软管+1个锥套+1个受油机 
VrAngle = zeros(22*3,1);
VrPos = zeros(22*3,1);

% 对于发送模型的视觉修正  全部在这里
% 由于这里只管发送 所以必须让前面模型在计算时也考虑这些修正，这样才能把各种计算都对上
hose_delta_pos = [0;0;0];                      % 视觉对齐 让软管都上升1m
drogue_delta_pos =[0;0;.04];                   % 调整锥套的位置 让它和最后一根软管对上 和软管一样先调整1m，再微调 其实就是 hose_delta_pos + [0.85;0;-0.15]
drogue_delta_angle = [0;0;0];                  % 调整锥套的角度 让它和最后一根软管的角度切合 rpy，pitch向上是正向下是负 [0;-8/180*pi;pi]
drogue_visual_pos = [-0.05;0;1.1];             % 这里要将锥套的位置反馈给前面做计算，要将锥套的视觉位置dr2tx+drogue_visual_pos=实际的锥套位置  
                                               % 方法是通过视觉识别得到的dr2cam(z)+cam2rc(z)+dr2tx(z)=rc2tx(z).这里dr2cam是准确的，只有dr2tx可变，所以修正到这里

% add
scale = 1;
for j = 1:21                        %前20为软管坐标数据，后1为软管平滑过渡处理
    if j == 1
        pX = [0, 0, 0]';            %软管起点
        pY = PosTb(3*j-2:3*j);      %软杆终点
                                    % 不用平滑的 直接用锥套的真实位置
    elseif j == 21                  %多加一段杆，做过渡
        pX = PosTb(3*j-5:3*j-3);
        pY = [PosTb(3*j-5)-0.7163*cos(8/180*pi),PosTb(3*j-4),PosTb(3*j-3)+0.7163*sin(8/180*pi)]';
    else
        pX = PosTb(3*j-5:3*j-3);
        pY = PosTb(3*j-2:3*j); 
    end
    
    pZ = (pX + pY)/2;                   %中点坐标

    %到VR中比例的缩放
    pZ = pZ * scale;
    
    vAxis = [0,0,-1]';                  %水平轴
    vTb = pY - pX;                      %杆的方向
    
    axis1 = null([vAxis';vTb']);        %获取垂直向量
    vRot = axis1(:,1)';                 %得到旋转轴
    
    if vRot(2) < 0
        vRot = -vRot;
    end
 
    yaw_xoz = asin(vTb(2) / sqrt(vTb(1)*vTb(1) + vTb(2)*vTb(2)+ vTb(3)*vTb(3)));
    pitch_z = pi - atan(vTb(3) / vTb(1));
%     pitch_z = atan(vTb(3) / vTb(1));
    roll = 0;   % 圆柱形hose，不用计算roll   
    VrAngle(3*j-2:3*j) = [yaw_xoz, pitch_z, roll];
    % 视觉对齐 让软管都上升hose_delta_posm
    VrPos(3*j-2:3*j) = [pZ(1);pZ(2);pZ(3)] + hose_delta_pos;
end
% add 发送的是受油机的位置
VrAngle(64:66)=[AttitudeRecei(1);AttitudeRecei(2);AttitudeRecei(3)];

pZ = Pos_rc2tx;
pZ = pZ * scale;
VrPos(3*22-2:3*22) = [pZ(1),pZ(2),pZ(3)]';


tmp1 = VrPos(1:60,:);                               % 软管位置
tmp2 = VrPos(61:63,:) + drogue_delta_pos;           % 锥套位置
tmp3 = VrPos(64:66,:) ;                             % 受油机位置 
tmp4 = VrAngle(1:60,:);                             % 软管角度
tmp5 = tmp4(58:60) + drogue_delta_angle;            % 锥套角度 使用的是最后一根软管的角度
tmp6 = VrAngle(64:66,:);                            % 受油机角度

tmp=[tmp1;tmp4;tmp2;tmp5;tmp3;tmp6];
y = tmp;

% 发送反馈给前面的锥套位置由于视觉上有差异，所以需要修正 但是实际上发送的是tmp2，并没有发送调整过的值 
Pos_dr2tx=tmp2+drogue_visual_pos;

== matlab function AirRefueling_Platform_IBVS/Tanker system/   ==
  data: u input; y output
function y = WindTurFromTank(u)
%#codegen

y = TankerVortexWindField(u);

== matlab function AirRefueling_Platform_IBVS/Hose-drogue system/DRdynamics/Hose-Drogue1/Calculate the Acceleration of the Links1/MATLAB Function2 ==
  data: t0 output size=1; T input; q input; t output
function [t0,t] = fcn(T,q)
% 由于编译报错所以用下面两行来替换第三行。
t = zeros(10,1);
t = inv(T)*q;
% t = T\q;
t0 = t(1);

== matlab function AirRefueling_Platform_IBVS/Hose-drogue system/DRdynamics/Hose-Drogue1/Calculate the Acceleration of the Links1/MATLAB Function3 ==
  data: t input; Q input; n input; m1 input; Mdr input; a output; N parameter; m0 parameter
function a = fcn(t,Q,n,m1,Mdr, N,m0)
a = zeros(3,N);
a(:,1) = (t(1)*n(:,1) - t(2)*n(:,2) + Q(:,1))/m1;
for i = 2:N-1
    a(:,i) = (t(i)*n(:,i) - t(i+1)*n(:,i+1) + Q(:,i))/m0;
end
a(:,N) = (t(N)*n(:,N) + Q(:,N))/(m0/2 + Mdr);                %注意最后一个节点的质量！！

== matlab function AirRefueling_Platform_IBVS/Hose-drogue system/DRdynamics/Hose-Drogue1/Calculate the Acceleration of the Links1/MATLAB Function4 ==
  data: n input; dn input; q output; Q input; m1 input; l1 input; ddl1 input; a0 input; N parameter; l0 parameter; m0 parameter
function q = fcn(n,dn,Q,m1,l1,ddl1,a0, N,l0,m0)

% n = 连杆的方向向量，想上为正 向量3*N
% Q = 连杆所受的合外力 向量3*N
% m = 连杆质量 向量1*N
% l = 连杆长度 向量1*N
% dl = 连杆长度的一阶导数 向量1*N
% ddl = 连杆长度的二阶导数 向量1*N
% a0 = 连接点的加速度 向量3*1

%%%%求张力t%%%%%%%%%%%%%%%%%%%%%%%%%%%%%%%%%%%%%%%%%%%%%%%%%%%%%%
q = zeros(N,1);
q(1,1) = m1*l1*dn(:,1)'*dn(:,1) - Q(:,1)'*n(:,1) + m1*a0'*n(:,1) - m1*ddl1;
q(2,1) = l0*dn(:,2)'*dn(:,2) + (1/m1*Q(:,1) - 1/m0*Q(:,2))'*n(:,2); % 可参考有关变长度连杆的《推导》
for i = 3:N
    q(i,1) = l0*dn(:,i)'*dn(:,i) + (1/m0*Q(:,i-1) - 1/m0*Q(:,i))'*n(:,i);
end

== matlab function AirRefueling_Platform_IBVS/Hose-drogue system/Collision Detection/MATLAB Function1 ==
  settings: updateMethod=DISCRETE
  data: Pos_pr input; F output; V_pr input; Pos_dr input; V_dr input; Mdr input; visual_err input
function F = fcn(Pos_pr,V_pr,Pos_dr,V_dr,Mdr,visual_err)
% 在x方向，椎管刚接触到锥套的时候，两者差是0.2m，完全进入时两者差是0.8
% 在z方向，椎管在锥套最下沿的时候，两者差是0.21m，在正中间的时候是0.12m 感觉这个不准
% error =z^2+y^2-x^2; 
% error<0 代表在圆锥里面
% 当x进入一定范围之内时，才能计算误差
% 当前位置减去定点的位置 相当于把定点放在了原点 x^2 = y^2 + z^2 （x<0）
% 分成xyz三个方向进行误差计算 
% x的范围[-0.2,0.45]  yz的范围相同,就是x一定时，半径时y=z=x对应的圆形的范围[-y,y]
% 给定了x之后 要判断两个 第一个是在这个圆形范围内，第二个是距离圆心的距
F = zeros(3,1);
% modify = [0.66;-0.1;0.645]*0+[0.7;-0.1;0.8]*0;
modify = visual_err;
% 是锥套位置-椎管位置 初始值是大于0的
x = Pos_dr(1) - Pos_pr(1)+ modify(1);
y = Pos_dr(2) - Pos_pr(2)+ modify(2);
% 椎管的z坐标要反一下 
z = Pos_dr(3) - Pos_pr(3)+ modify(3);
Vel_relative = V_pr - V_dr;

error =z^2+y^2-x^2; 
Kp_p = 100;
Kp_v = 50; 
persistent f;     
if(isempty(f))
    f=[0;0;0];
end
if x<0.05
%     F(1)= 1000 * Mdr * (-x) + 500 * Mdr * (Vel_relative(1));
%     % y方向的
%     F(2)= 1000 * Mdr * (-y) + 500 * Mdr * (Vel_relative(2));
%     % z方向的
%     F(3)= 1500 * Mdr * (-z) + 500 * Mdr * (Vel_relative(3));
    if x>-0.05
    F(1)= 100 * Mdr * (-x) + 1 * Mdr * (Vel_relative(1));
    % y方向的
    F(2)= 20 * Mdr * (-y) + 2 * Mdr * (Vel_relative(2));
    % z方向的
    F(3)= 20 * Mdr * (-z) + 2 * Mdr * (Vel_relative(3));
    f = F;
    else
        F=f;
    end
end
% F = zeros(3,1);

== matlab function AirRefueling_Platform_IBVS/Hose-drogue system/MATLAB Function ==
  data: P_dr input; P_link10 input; P_hose_dr output
function P_hose_dr = fcn(P_dr,P_link10)
% P_link20=zeros(3,20);
% P_link20(:,1) = P_link10(:,1)/2;
% P_link20(:,2) = P_link10(:,1);
% P_link20(:,3) = (P_link10(:,2)+P_link10(:,1))/2;
% P_link20(:,4) = P_link10(:,2);
% P_link20(:,5) = (P_link10(:,3)+P_link10(:,2))/2;
% P_link20(:,6) = P_link10(:,3);
% P_link20(:,7) = (P_link10(:,4)+P_link10(:,3))/2;
% P_link20(:,8) = P_link10(:,4);
% P_link20(:,9) = (P_link10(:,5)+P_link10(:,4))/2;
% P_link20(:,10) = P_link10(:,5);
% P_link20(:,11) = (P_link10(:,6)+P_link10(:,5))/2;
% P_link20(:,12) = P_link10(:,6);
% P_link20(:,13) = (P_link10(:,7)+P_link10(:,6))/2;
% P_link20(:,14) = P_link10(:,7);
% P_link20(:,15) = (P_link10(:,8)+P_link10(:,7))/2;
% P_link20(:,16) = P_link10(:,8);
% P_link20(:,17) = (P_link10(:,9)+P_link10(:,8))/2;
% P_link20(:,18) = P_link10(:,9);
% P_link20(:,19) = (P_link10(:,10)+P_link10(:,9))/2;
% P_link20(:,20) = P_link10(:,10);
% %P_link20(:,20) = P_dr;
% P_link20_V60 = reshape(P_link20,60,1);


%% 

x = P_link10(1,:);
y = P_link10(2,:);
z = P_link10(3,:);
n=length(x)-1;% B样条曲线有n+1个控制点
k=4;% 三次B样条，因此阶数=次数+1

% 用于储存生成的点
X=[];
Y=[];
Z=[];

Nik_u=zeros(1,n+1);% 用于储存基函数
nodevector=U_quasi_uniform(n,k);% 生成节点向量

for u=0:0.01:1-0.01% 循环次数决定组成B样条曲线点的总数量
    for j=1:n+1% 生成Bi,3这一系列基函数
        Nik_u(j)=BaseFunction(j,k,u,nodevector);
    end
    % 由于B样条曲线具有局部支撑性，因此只有u周围一定区间会参与到计算
    X=[X,x*Nik_u'];
    Y=[Y,y*Nik_u'];
    Z=[Z,z*Nik_u'];
end
% 根据三次B样条插值的结果得到20根管子的位置
P_link20=zeros(3,20);
index = 1;
for i=1:length(X)/20:100
    P_link20(:,index)=[X(i),Y(i),Z(i)];
    index = index+1;
end

P_link20_V60 = reshape(P_link20,60,1);
% 再将锥套的真实位置传过去 此时是63*1(20根管子+1个锥套)的向量 前面60个是软管 最后三个是锥套
P_hose_dr = [P_link20_V60;P_dr];

== matlab function AirRefueling_Platform_IBVS/Receiver System/Controller/IBVS Conroller ==
  data: Z input; ex input; ey input; u_vcz output; u_vcy output; u_vcx output; F16State input
function [u_vcz,u_vcy,u_vcx] = fcn(Z,ex,ey, F16State)

%receiver和camer之间的距离为d_cam_rc = [4.7;0.54;-1.45]- [0;0;2.05];
L_x = 4.7;
L_y = 0.54;
L_z = -3.5;

ey = -ey;%坐标系转换需要变号。

%% 对接成功，参数也对。
% Z_d = 2.0;
Z_d = -1;

% kz = 0.3;
% ky = 1;
% kx = 1;
kz = 2; %kz对应书中的k3
ky = 10; %ky对应书中的k2
kx = 10; %kx对应书中的k1


k1 = 3; k2 = 1;%k1对应书中的k4,k2对应书中的k5
%F16State(10,1)是p，F16State(11,1)是q，F16State(12,1)是r。在刘浩论文中，相机安装在锥管前端，receiver和camer之间的距离为d_pr_rc = [6.06;0.54;-0.86];
% u_vcz = kz*(Z-Z_d)-k1*(abs(ex)/abs(Z))-k2*(abs(ey)/abs(Z))-F16State(10,1)*0.86+F16State(12,1)*0.54;
% u_vcy = ky*(ey-0)-F16State(10,1)*0.54+F16State(11,1)*6.06;
% u_vcx = kx*(ex-0)-F16State(12,1)*6.06+F16State(10,1)*0.86;

u_vcz = kz*(Z-Z_d)-k1*(abs(ex)/abs(Z))-k2*(abs(ey)/abs(Z))+F16State(10,1)*L_z+F16State(12,1)*L_x;
u_vcy = ky*(ey-0)-F16State(10,1)*L_y+F16State(11,1)*L_x;
u_vcx = kx*(ex-0)-F16State(12,1)*L_x+F16State(10,1)*L_z;




%% 利用迭代学习的前向速度控制，使用图像误差缩小横竖误差，这里可以对接成功。
% ky = 3;
% u_vcy = ky*(ey-(0.5));
% kx = 1;
% u_vcx = kx*(ex-0);



%% 第二次控制实验：加入头波的影响后，当前参数也可以完成对接。此时头波大小在仿真里为1倍。
% %10倍头波在此参数下只能接近，不能对接成功。
% Z_d = 2.0;
% kz = 0.5;
% ky = 5;
% 
% 
% k1 = 3; k2 = 1;
% % u_vcz = kz*(Z-Z_d)-k1*(abs(ex))-k2*(abs(ey));
% u_vcz = kz*(Z-Z_d)-k1*(abs(ex)/abs(Z))-k2*(abs(ey)/abs(Z));
% u_vcy = ky*(ey-0);
% 
% kx = 1.6;
% u_vcx = kx*(ex-0);


% Z_d = 2.0;
% kz = 0.5;
% ky = 2;
% 
% k1 = 3; k2 = 1;
% % u_vcz = kz*(Z-Z_d)-k1*(abs(ex))-k2*(abs(ey))-F16State(10,1)*0.86+F16State(12,1)*0.54;
% u_vcz = kz*(Z-Z_d)-k1*(abs(ex)/abs(Z))-k2*(abs(ey)/abs(Z))-F16State(10,1)*0.86+F16State(12,1)*0.54;
% u_vcy = ky*(ey-0)-F16State(10,1)*0.54+F16State(11,1)*6.06;
% 
% kx = 1;
% u_vcx = kx*(ex-0)-F16State(12,1)*6.06+F16State(10,1)*0.86;

== matlab function AirRefueling_Platform_IBVS/Hose-drogue system/DRdynamics/Hose-Drogue1/Calculate the External Force of the Links/MATLAB Function ==
  data: vr input; n input; Ref output; radius input; viscosity input; Cf output; Red output; Cd output; N parameter
function [Ref, Cf, Red, Cd] = C(vr,n,radius,viscosity, N)
% 计算雷诺数以及相应的摩擦系数Cf和压差系数Cd

% 单杆的速度、方向等用3*1的列向量表示
% vr = 连杆相对风速度 向量3*N
% n = 连杆的方向向量，想上为正 向量3*N
% viscosity  = 动粘度系数
% radius = 连杆半径

%——计算雷诺数———————————————————————————
cosa = zeros(1,N);
sina = zeros(1,N);
Ref = zeros(1,N);
Red = zeros(1,N);
for i = 1:N
    if norm(vr(:,i)) ~= 0
        cosa(i) = vr(:,i)'*n(:,i)/norm(vr(:,i));
        sina(i) = sqrt(1-cosa(i)^2);
        if sina(i) ~= 0
            Ref(i) = (pi*radius/viscosity)*norm(vr(:,i))/sina(i);
        else
            Ref(i) = 10^11;
        end
        Red(i) = norm(vr(:,i))*2*radius/viscosity;
    end
end

%——计算气动系数——————————————————————————
Cf = zeros(1,N);
Cd = zeros(1,N);
for i = 1:N
    %%%%Cf表%%%%%%%%%%%%%%%%%%%%%%%%
    if Ref(i)<=10^-2
        Cf(i) = 0;    %注意这里有改动
    elseif Ref(i)>10^-2 && Ref(i)<=10^4
        Cf(i) = 4.6409*Ref(i)^-0.6667;
    elseif Ref(i)>10^4 && Ref(i)<=10^10
        Cf(i) = 0.0464*Ref(i)^-0.1667;
    elseif Ref(i)>10^10
        Cf(i) = 0.001;
    end
    %%%%Cd表%%%%%%%%%%%%%%%%%%%%%%%%%
    if Red(i)<=10^-2
        Cd(i) = 0;   %注意这里有改动
    elseif Red(i)>10^-2 && Red(i)<=1
        Cd(i) = 10*Red(i)^-0.801;
    elseif Red(i)>1 && Red(i)<=180
        Cd(i) = 10*Red(i)^-0.4083;
    elseif Red(i)>180 && Red(i)<=4*10^5
        Cd(i) = 1.2;
    elseif Red(i)>4*10^5 && Red(i)<=4*10^6
        Cd(i) = 0.002128*Red(i)^0.3522;
    elseif Red(i)>4*10^6
        Cd(i) = 0.45;
    end
end

== matlab function AirRefueling_Platform_IBVS/Hose-drogue system/DRdynamics/Hose-Drogue1/Calculate the External Force of the Links/MATLAB Function1 ==
  data: vr input; Q output; n input; Cf input; Cd input; l1 input; density input; radius input; Rdr input; Cdr input; Mdr input; rou input; p input; Fb input; Df_mid output; Dd_mid output; Df output; Dd output; D output; Ddr output; N parameter; l0 parameter; fen_norm output; fen output
function [Q, Df_mid, Dd_mid, Df, Dd, D, Ddr, fen_norm, fen] = ExternalForce(vr,n,Cf,Cd,l1,density,radius,Rdr,Cdr,Mdr,rou,p,Fb, N,l0)

% 计算每根连杆的合外力

% 单杆的速度、方向等用3*1的列向量表示
% l = 每根连杆的长度，注意这里要做成变长的 向量
% vr = 连杆相对风速度 向量3*N
% n = 连杆的方向向量，想上为正 向量3*N
% viscosity  = 大气动粘度系数
% density = 大气密度
% radius = 连杆半径
% r_dr = 锥套伞冠半径
% rou = 连杆的线密度

% Cdr = 锥套的阻力系数
% Rdr = 锥套伞冠半径
% Mdr = 锥套质量

%——求气动力————————————————————————————
Df_mid = zeros(1,N);
Dd_mid = zeros(1,N);
Df = zeros(3,N);
Dd = zeros(3,N);
D = zeros(3,N);
vn = zeros(3,N);
for i = 1:N
    if i == 1
        Df_mid(i) = density*pi*radius*l1*Cf(i)*(vr(:,i)'*n(:,i))^2;
    else
        Df_mid(i) = density*pi*radius*l0*Cf(i)*(vr(:,i)'*n(:,i))^2;
    end
    if vr(:,i)'*n(:,i)>0   % 这里可能有符号问题，万一之后还是出现杂乱的情况，要注意这里
        Df(:,i) = Df_mid(i)*n(:,i);
    else
        Df(:,i) = - Df_mid(i)*n(:,i);
    end
    % 当杆的方向迎着风的时候，摩擦阻力延杆反向
    % 当杆的方向顺着风的时候，摩擦阻力延杆正向
    
    vn(:,i) = vr(:,i)-(vr(:,i)'*n(:,i))*n(:,i); 
    if i == 1
        if norm(vn(:,i)) ~= 0
            Dd_mid(i) = density*radius*l1*Cd(i)*norm(vn(:,i))^2;
            Dd(:,i) = - Dd_mid(i)*vn(:,i)/norm(vn(:,i));
        else
            Dd(:,i) = [0;0;0];
        end
    else
        if norm(vn(:,i)) ~= 0
            Dd_mid(i) = density*radius*l0*Cd(i)*norm(vn(:,i))^2;
            Dd(:,i) = - Dd_mid(i)*vn(:,i)/norm(vn(:,i));
        else
            Dd(:,i) = [0;0;0];
        end
    end
    % 无论连杆与相对速度的角度关系如何，压差阻力总是顺着风的方向的
        
    D(:,i) = Df(:,i) + Dd(:,i);
end

if vr(:,N)'*vr(:,N) ~= 0
    Ddr = - 1/2*density*vr(:,N)'*vr(:,N)*(pi*Rdr^2)*(Cdr)* vr(:,N)/norm(vr(:,N));
else
    Ddr = [0;0;0];
end
%%%%%%%%%%%%%%%%%%%%%%%%%%%%%%%%%%%%%%%%%%%%%%%%%%%%%%%%%%%%%%%%

% %%%%计算恢复力%%%%%%%%%%%%%%%%%%%%%%
do = 1; % 连杆外径
di = 0.84; % 连杆内径
E = 589.67; % 弹性系数 数量级可能有问题
K = E*pi/8*(do^4 - di^4);
fen_norm = zeros(1,N);
fen = zeros(3,N);
for i = 2:N-1
    n0mid = (p(:,i-1) - p(:,i+1))/norm(p(:,i-1) - p(:,i+1));
    if abs(norm(n(:,i-1)'*n(:,i))-1) ~= 0;
        gama1 = n(:,i-1)'*n0mid;
        gama2 = n(:,i)'*n0mid;
        if norm(gama1) >= 1
            gama1 = gama1/abs(gama1);
        end
        if norm(gama2) >= 1
            gama2 = gama2/abs(gama2);
        end
            
        fen_norm(i) = K*(acos(gama1) + acos(gama2))/norm(p(:,i-1) - p(:,i+1))^2;
        fen(:,i) = fen_norm(i)*((n(:,i)'*n0mid*n0mid - n(:,i))*1e3)/norm((n(:,i)'*n0mid*n0mid - n(:,i))*1e3);
    end
end
%%%%%%%%%%%%%%%%%%%%%%%%%%%%%%%%%%%%%%

% %%%%计算合外力%%%%%%%%%%%%%%%%%%%%%%?
% Q = zeros(3,N);
% for i = 1:N-1
%     Q(:,i) = [0;0;m*g] + 1/2*(D(:,i)+D(:,i+1));
% end
% Q(:,N) = [0;0;(m+Mdr)*g] + 1/2*D(:,N) + Ddr;
Q = zeros(3,N);
Q(:,1) = [0;0;l1*rou*9.8] + 1/2*(D(:,1)+D(:,2)) + fen(:,1);
for i = 2:N-1
    Q(:,i) = [0;0;l0*rou*9.8] + 1/2*(D(:,i)+D(:,i+1)) + fen(:,i);
end
Q(:,N) = [0;0;(l0/2*rou + Mdr)*9.8] + 1/2*D(:,N) + Ddr + Fb;        %注意最后一个节点的质量
% 这里删掉了锥套的受力（Bow wave），后面再处理
% %%%%%%%%%%%%%%%%%%%%%%%%%%%%%%%%

== matlab function AirRefueling_Platform_IBVS/Hose-drogue system/DRdynamics/Hose-Drogue1/Calculate the Orientation of the Links1/MATLAB Function ==
  data: nd1 output; nd2 output; theta1 input; n output; theta2 input; N parameter
function [nd1,nd2,n] = fcn(theta1,theta2, N)
% theta1,theta2 向量1*n
n = zeros(3,N);
nd1 = zeros(3,N);
nd2 = zeros(3,N);

for i = 1:N
    n(:,i) = [cos(theta1(i))*cos(theta2(i)); sin(theta2(i)); -sin(theta1(i))*cos(theta2(i))];
    nd1(:,i) = [-sin(theta1(i))*cos(theta2(i)); 0; -cos(theta1(i))*cos(theta2(i))];
    nd2(:,i) = [-cos(theta1(i))*sin(theta2(i)); cos(theta2(i)); sin(theta1(i))*sin(theta2(i))];
end
